simulink model "simulacion_Ejercicio1_examen_7_1_2020"  (R2024a)
settings: Solver=FixedStepAuto  StartTime=0.0  StopTime=15  FixedStep=0.001  RelTol=1e-3
values from neighbouring files (symbols this model uses):
  a_adelanto = y + Pd1_real    [Ejercicio1_examen_7_1_2020.m]
  b_adelanto = 1    [Ejercicio1_examen_7_1_2020.m]
  final_escalon = 1    [Ejercicio1_examen_7_1_2020.m]
  Mp = 20.788 / 100    (= 0.20788)    [Ejercicio1_examen_7_1_2020.m]
undefined symbols (not defined in the file or in its folder): K_rlocfind
libraries: simulink x1
settings Model: Creator=david  LastModifiedBy=david

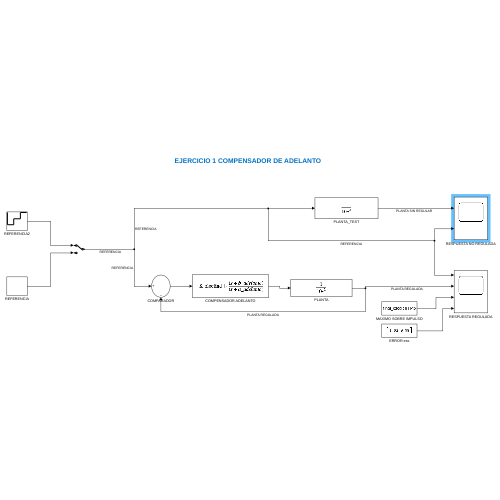
[thumbnail: Simulink's stored preview of the top-level diagram]
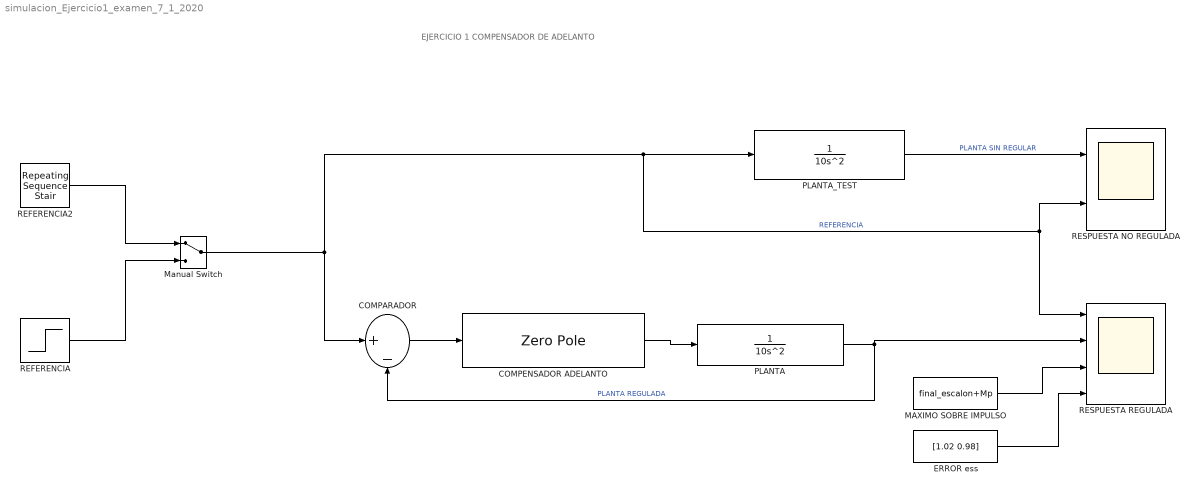
== system simulacion_Ejercicio1_examen_7_1_2020 ==
  note: EJERCICIO 1 COMPENSADOR DE ADELANTO
  COMPARADOR : Sum  Inputs=|+-
  COMPENSADOR ADELANTO : ZeroPole  Zeros=[-b_adelanto]  Poles=[-a_adelanto]  Gain=[K_rlocfind]
  ERROR ess : Constant  Value=[1.02 0.98]
  MAXIMO SOBRE IMPULSO : Constant  Value=final_escalon+Mp
  Manual Switch : ManualSwitch
  PLANTA : TransferFcn  Denominator=[10 0 0]
  PLANTA_TEST : TransferFcn  Denominator=[10 0 0]
  REFERENCIA : Step  After=final_escalon  SampleTime=0
  REFERENCIA2 : simulink/Sources/Repeating Sequence Stair  OutValues=[1 2 3]  tsamp=5  OutMin=[]  OutMax=[]  OutDataTypeStr=double  OutputDataTypeScalingMode=double  OutDataType=fixdt(0,8)  ConRadixGroup=Best Precision: Vector-wise  OutScaling=2^-12
  RESPUESTA NO REGULADA : Scope  NumInputPorts=2
  RESPUESTA REGULADA : Scope  NumInputPorts=4
  wires:
  Manual Switch/1 -> COMPARADOR/1, PLANTA_TEST/1, RESPUESTA NO REGULADA/2, RESPUESTA REGULADA/1  "REFERENCIA"
  COMPARADOR/1 -> COMPENSADOR ADELANTO/1
  COMPENSADOR ADELANTO/1 -> PLANTA/1
  PLANTA/1 -> RESPUESTA REGULADA/2, COMPARADOR/2  "PLANTA REGULADA"
  PLANTA_TEST/1 -> RESPUESTA NO REGULADA/1  "PLANTA SIN REGULAR"
  MAXIMO SOBRE IMPULSO/1 -> RESPUESTA REGULADA/3
  ERROR ess/1 -> RESPUESTA REGULADA/4
  REFERENCIA2/1 -> Manual Switch/1
  REFERENCIA/1 -> Manual Switch/2
